simulink model "TwoSwitchFlybackConv"  (R2021b)
settings: Solver=ode4  StartTime=0.0  StopTime=1.425e-3  FixedStep=5e-10  RelTol=1e-3
values from neighbouring files (symbols this model uses):
  C2 = D2/fs*(Vc2-Vbat2)/Rout2/delVc2    (= 2.79316389763e-06)    [Script.m]
  fs = 250e3    (= 250000)    [Script.m]
  Gcinf2 = (abs(evalfr(Tuiind2,1i*2*pi*fc)))/sqrt(1+(wLv2/2/pi/fc)^2)/abs(evalfr(Gfilter,1i*2*pi*fc))    [Script.m]
  Lm2 = Vc2*Dp2/delIlm2/fs    (= 0.00253168682241)    [Script.m]
  Rin2 = 100e-3    (= 0.1)    [Script.m]
  Rout2 = 3*Rin2    (= 0.3)    [Script.m]
  Rsense2 = 5/0.1    (= 50)    [Script.m]
  Vbat2 = 3*3.7    (= 11.1)    [Script.m]
  Vin2 = 3.7    [Script.m]
  Vm = 5    [Script.m]
  wLv2 = 2*pi*fc*tan(60*pi/180)    [Script.m]
  wpfilter2 = 2*pi*10e3    (= 62831.8530718)    [Script.m]
libraries: spsCurrentMeasurementLib x6, spsVoltageMeasurementLib x6, spsSeriesRLCBranchLib x4, spsMosfetLib x3, spsDiodeLib x2, spsDCVoltageSourceLib x2, spsLinearTransformerLib x1, simulink x1, spspowerguiLib x1
settings Model: SimulationMode=rapid-accelerator  Creator=Aditya Bhalotia  LastModifiedBy=ee3210698
settings DebuggingCC: UnconnectedInputMsg=none  UnconnectedOutputMsg=none  UnconnectedLineMsg=none
settings RTWCC: DLArmComputeVersion=20.02.1

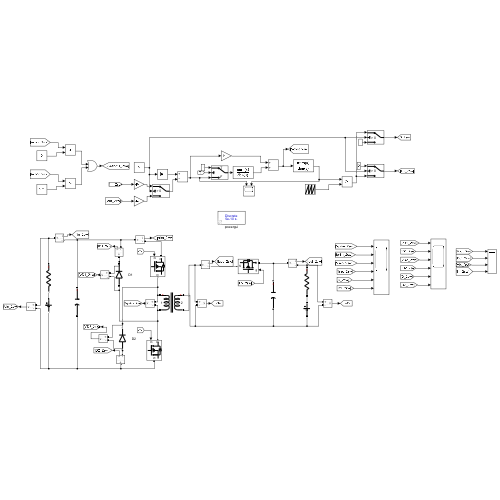
[thumbnail: Simulink's stored preview of the top-level diagram]
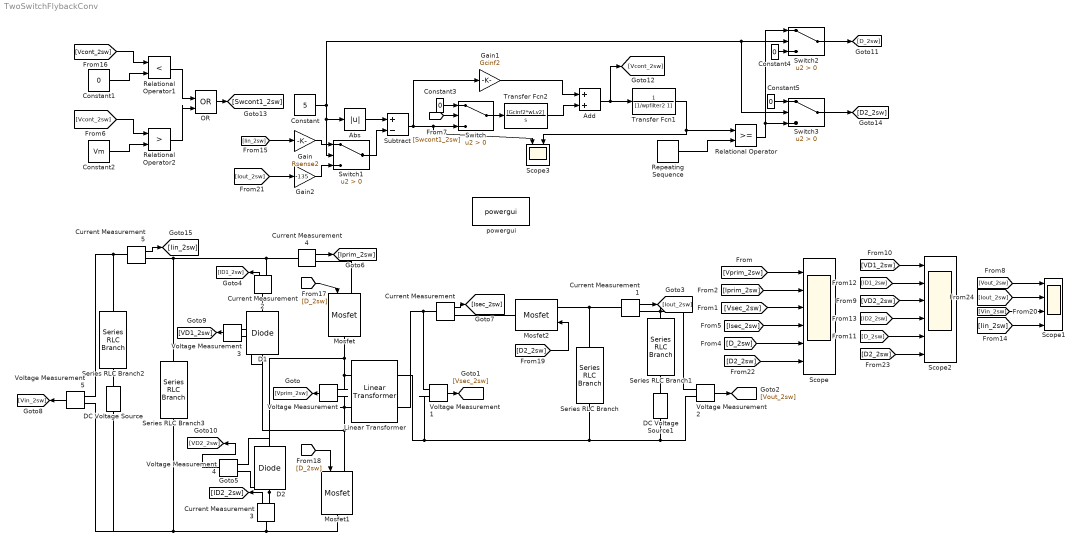
== system TwoSwitchFlybackConv ==
  Abs : Abs
  Add : Sum
  Constant : Constant  Value=5
  Constant{1,3..5} (4 alike) : Constant  Value=0
  Constant2 : Constant  Value=Vm
  Current Measurement{,1..5} (6 alike) : spsCurrentMeasurementLib/Current Measurement  PhasorSimulation=off  OutputType=Complex  PSBequivalent=0
  D1 : spsDiodeLib/Diode  Ron=0.001  Lon=0  Vf=0  IC=0  UseSnubber=0  Rs=inf  Cs=inf  Measurements=off
  D2 : spsDiodeLib/Diode  Ron=0.001  Lon=0  Vf=0  IC=0  UseSnubber=0  Rs=inf  Cs=inf  Measurements=off
  DC Voltage Source : spsDCVoltageSourceLib/DC Voltage Source  Amplitude=Vin2  Measurements=None
  DC Voltage Source1 : spsDCVoltageSourceLib/DC Voltage Source  Amplitude=Vbat2  Measurements=None
  Gain : Gain  Gain=Rsense2
  Gain1 : Gain  Gain=Gcinf2
  Gain2 : Gain  Gain=-135
  Linear Transformer : spsLinearTransformerLib/Linear Transformer  UNITS=SI  NominalPower=[ 200 fs ]  winding1=[10 0 0]  winding2=[40 0 0]  ThreeWindings=off  winding3=[3.15e+05 0.7938 0.084225]  RmLm=[inf Lm2]  Measurements=None  DataType=on
  Mosfet : spsMosfetLib/Mosfet  Ron=0.001  Lon=0  Rd=0.001  Vfd=0  IC=0  Rs=1e9  Cs=inf  Measurements=off
  Mosfet1 : spsMosfetLib/Mosfet  Ron=0.1  Lon=0  Rd=0.01  Vfd=0  IC=0  Rs=1e9  Cs=inf  Measurements=off
  Mosfet2 : spsMosfetLib/Mosfet  Ron=0.1  Lon=0  Rd=0.01  Vfd=0  IC=0  Rs=1e9  Cs=inf  Measurements=off
  OR : Logic  Operator=OR  IconShape=distinctive  AllPortsSameDT=off  OutDataTypeStr=boolean
  Relational Operator : RelationalOperator  OutDataTypeStr=boolean  RndMeth=Simplest
  Relational Operator1 : RelationalOperator  Operator=<  OutDataTypeStr=boolean  RndMeth=Simplest
  Relational Operator2 : RelationalOperator  Operator=>  OutDataTypeStr=boolean  RndMeth=Simplest
  Repeating Sequence : simulink/Sources/Repeating Sequence  rep_seq_t=[0 1/fs]  rep_seq_y=[0 Vm]
  Scope : Scope  NumInputPorts=6
  Scope1 : Scope  NumInputPorts=4
  Scope2 : Scope  NumInputPorts=6
  Scope3 : Scope  NumInputPorts=2
  Series RLC Branch : spsSeriesRLCBranchLib/Series RLC Branch  LConnTagsString=__new0  RConnTagsString=__new0  BranchType=C  Resistance=1  Inductance=1e-3  SetiL0=off  InitialCurrent=0  Capacitance=C2  Setx0=off  InitialVoltage=0  Measurements=None
  Series RLC Branch1 : spsSeriesRLCBranchLib/Series RLC Branch  LConnTagsString=__new0  RConnTagsString=__new0  BranchType=R  Resistance=Rout2  Inductance=1e-3  SetiL0=off  InitialCurrent=0  Capacitance=1e-6  Setx0=off  InitialVoltage=0  Measurements=None
  Series RLC Branch2 : spsSeriesRLCBranchLib/Series RLC Branch  LConnTagsString=__new0  RConnTagsString=__new0  BranchType=R  Resistance=Rin2  Inductance=1e-3  SetiL0=off  InitialCurrent=0  Capacitance=1e-6  Setx0=off  InitialVoltage=0  Measurements=None
  Series RLC Branch3 : spsSeriesRLCBranchLib/Series RLC Branch  LConnTagsString=__new0  RConnTagsString=__new0  BranchType=C  Resistance=1  Inductance=1e-3  SetiL0=off  InitialCurrent=0  Capacitance=C2*3  Setx0=off  InitialVoltage=0  Measurements=None
  Subtract : Sum  Inputs=+-
  Switch{,1..3} (4 alike) : Switch  Criteria=u2 > Threshold
  Transfer Fcn1 : TransferFcn  Denominator=[1/wpfilter2 1]
  Transfer Fcn2 : TransferFcn  Numerator=[Gcinf2*wLv2]  Denominator=[1 0]
  Voltage Measurement{,1..5} (6 alike) : spsVoltageMeasurementLib/Voltage Measurement  PhasorSimulation=off  OutputType=Complex  PSBequivalent=0
  powergui : spspowerguiLib/powergui  Priority=1  SimulationMode=Discrete  SampleTime=5e-10  frequency=60  Iterations=50  frequencyindice=0  Pbase=100e6  ErrMax=1e-4  UnitsV=kV  UnitsW=MW  buscounter=0  FunctionMessages=off  echomessages=off  EnableUseOfTLC=off  CurrentSourceSwitches=off  DisableSnubberDevices=off  DisableRonSwitches=off  DisableVfSwitches=off  DisplayEquations=off  AutomaticDiscreteSolvers=off  SolverType=Tustin/Backward Euler (TBE)  Interpol=off  ExternalGateDelay=off  methode=off  Ts=100  x0status=blocks  SPID=on  SwTol=0  HookPort=off  NonlinearTolerance=1e-4  nMaxIteration=100  ContinueOnMaxIteration=off  RestoreLinks=warning  ResistiveCurrentMeasurement=off  Frange=[0:2:500]  Ylog=off  Xlog=on  ShowGrid=off  save=off  variable=ZData  structure=0  ZoomFFT=off  StartTime=0.0  cycles=1  DisplayStyle=1  fundamental=60  FreqAxis=off  MaxFrequency=1000  frequencyindicesteady=1  RmsSteady=1  display=off
  wires:
  [D_2sw] -> Mosfet1/1
  [D_2sw] -> Mosfet/1
  Voltage Measurement/1 -> [Vprim_2sw]
  Voltage Measurement1/1 -> [Vsec_2sw]
  Current Measurement2/1 -> [ID1_2sw]
  Current Measurement3/1 -> [ID2_2sw]
  Current Measurement4/1 -> [Iprim_2sw]
  Current Measurement/1 -> [Isec_2sw]
  Voltage Measurement2/1 -> [Vout_2sw]
  [Vprim_2sw] -> Scope/1
  [Iprim_2sw] -> Scope/2
  [Vsec_2sw] -> Scope/3
  [Isec_2sw] -> Scope/4
  [D_2sw] -> Scope/5
  [Vout_2sw] -> Scope1/1
  Voltage Measurement3/1 -> [VD1_2sw]
  Voltage Measurement4/1 -> [VD2_2sw]
  [VD1_2sw] -> Scope2/1
  [ID2_2sw] -> Scope2/4
  [D_2sw] -> Scope2/5
  [ID1_2sw] -> Scope2/2
  [VD2_2sw] -> Scope2/3
  Constant4/1 -> Switch2/3
  Switch1/1 -> Subtract/2
  Constant5/1 -> Switch3/1
  Abs/1 -> Subtract/1
  [Iout_2sw] -> Gain2/1
  Constant1/1 -> Relational Operator1/2
  [Vcont_2sw] -> Relational Operator2/1
  Switch3/1 -> [D2_2sw]
  [Vcont_2sw] -> Relational Operator1/1
  Constant2/1 -> Relational Operator2/2
  Gain2/1 -> Switch1/3
  Transfer Fcn2/1 -> Add/2
  Gain1/1 -> Add/1
  OR/1 -> [Swcont1_2sw]
  Switch/1 -> Transfer Fcn2/1
  [Swcont1_2sw] -> Switch/2
  Repeating Sequence/1 -> Relational Operator/2
  Switch2/1 -> [D_2sw]
  Subtract/1 -> Switch/3, Scope3/1, Gain1/1
  Relational Operator1/1 -> OR/1
  Relational Operator/1 -> Switch2/1, Switch3/3
  Relational Operator2/1 -> OR/2
  Transfer Fcn1/1 -> Scope3/2, Relational Operator/1
  Constant/1 -> Switch1/2, Abs/1, Switch3/2, Switch2/2
  Add/1 -> Transfer Fcn1/1, [Vcont_2sw]
  Gain/1 -> Switch1/1
  Constant3/1 -> Switch/1
  [D2_2sw] -> Mosfet2/1
  [Iin_2sw] -> Gain/1
  Voltage Measurement5/1 -> [Vin_2sw]
  [Vin_2sw] -> Scope1/3
  [D2_2sw] -> Scope/6
  [D2_2sw] -> Scope2/6
  Current Measurement5/1 -> [Iin_2sw]
  Current Measurement1/1 -> [Iout_2sw]
  [Iin_2sw] -> Scope1/4
  [Iout_2sw] -> Scope1/2
  connections:
  Series RLC Branch3/LConn1 -- Current Measurement5/RConn1 -- Current Measurement2/RConn1 -- Current Measurement4/LConn1
  Voltage Measurement4/LConn1 -- D2/RConn1 -- Mosfet/RConn1 -- Voltage Measurement/LConn1 -- Linear Transformer/LConn1
  Linear Transformer/LConn2 -- Voltage Measurement/LConn2 -- Voltage Measurement3/LConn2 -- D1/LConn1 -- Mosfet1/LConn1
  Mosfet1/RConn1 -- Current Measurement3/LConn1 -- Voltage Measurement5/LConn2 -- DC Voltage Source/LConn1 -- Series RLC Branch3/RConn1
  Linear Transformer/RConn1 -- Voltage Measurement1/LConn2 -- Series RLC Branch/RConn1 -- DC Voltage Source1/LConn1 -- Voltage Measurement2/LConn2
  Series RLC Branch1/LConn1 -- Current Measurement1/RConn1 -- Voltage Measurement2/LConn1
  Linear Transformer/RConn2 -- Current Measurement/LConn1 -- Voltage Measurement1/LConn1
  Current Measurement/RConn1 -- Mosfet2/RConn1
  Series RLC Branch2/RConn1 -- DC Voltage Source/RConn1
  Current Measurement2/LConn1 -- D1/RConn1 -- Voltage Measurement3/LConn1
  Current Measurement3/RConn1 -- D2/LConn1 -- Voltage Measurement4/LConn2
  Current Measurement4/RConn1 -- Mosfet/LConn1
  DC Voltage Source1/RConn1 -- Series RLC Branch1/RConn1
  Voltage Measurement5/LConn1 -- Current Measurement5/LConn1 -- Series RLC Branch2/LConn1
  Mosfet2/LConn1 -- Current Measurement1/LConn1 -- Series RLC Branch/LConn1
